simulink model "TASK_5"  (R2018a)
settings: Solver=VariableStepAuto  StartTime=0.0  StopTime=10.0  RelTol=1e-3
libraries: simulink x2
settings Model: Creator=User  LastModifiedBy=User

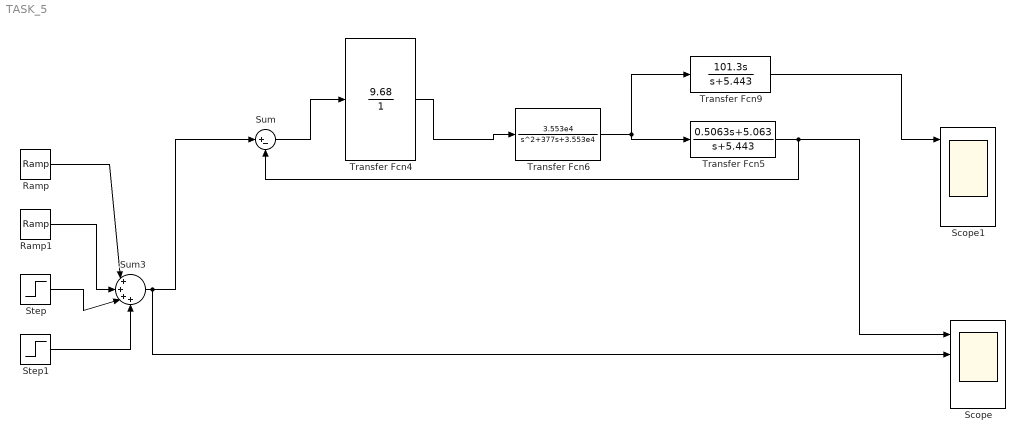
== system TASK_5 ==
  Ramp : simulink/Sources/Ramp  slope=63.158  start=1  InitialOutput=0
  Ramp1 : simulink/Sources/Ramp  slope=-63.158  start=1.23758  InitialOutput=0
  Scope : Scope  NumInputPorts=4
  Scope1 : Scope  NumInputPorts=4
  Step : Step  Time=0  After=5  SampleTime=0
  Step1 : Step  Time=5  After=-15  SampleTime=0
  Sum : Sum  Inputs=|+-
  Sum3 : Sum  Inputs=|++++
  Transfer Fcn4 : TransferFcn  Numerator=[9.68]  Denominator=[1]
  Transfer Fcn5 : TransferFcn  Numerator=[0.5063 5.063]  Denominator=[1 5.443]
  Transfer Fcn6 : TransferFcn  Numerator=[0 0 3.553e4]  Denominator=[1 377 3.553e4]
  Transfer Fcn9 : TransferFcn  Numerator=[101.3 0]  Denominator=[1 5.443]
  wires:
  Step/1 -> Sum3/3
  Transfer Fcn4/1 -> Transfer Fcn6/1
  Transfer Fcn5/1 -> Scope/1, Sum/2
  Sum/1 -> Transfer Fcn4/1
  Transfer Fcn9/1 -> Scope1/1
  Step1/1 -> Sum3/4
  Transfer Fcn6/1 -> Transfer Fcn5/1, Transfer Fcn9/1
  Ramp1/1 -> Sum3/2
  Ramp/1 -> Sum3/1
  Sum3/1 -> Scope/2, Sum/1
